simulink model "KP_sim"  (R2024b)
settings: Solver=VariableStepAuto  StartTime=0.0  StopTime=50  MaxStep=1e-3  RelTol=1e-3
values from neighbouring files (symbols this model uses):
  A = amplitudeValues(amplitudeIndex)    [KP_grid_results_generation.m]
  frequencyHz = frequencyValues(frequencyIndex)    [KP_grid_results_generation.m]
  x0 = [initialAngle; initialAngularVelocity]    [KP_grid_results_generation.m]
settings Model: Creator=Pedro  LastModifiedBy=Pedro

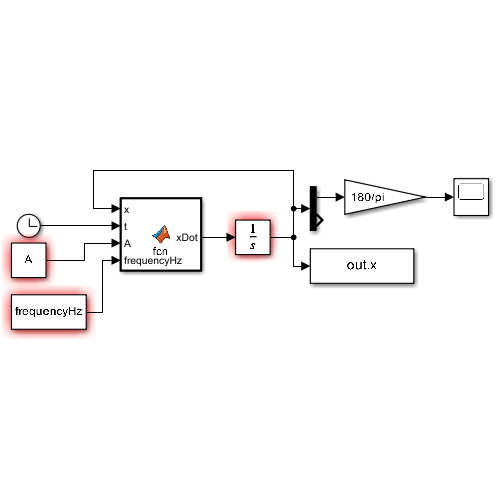
[thumbnail: Simulink's stored preview of the top-level diagram]
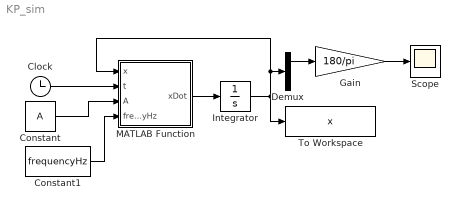
== system KP_sim ==
  Clock : Clock
  Constant : Constant  Value=A
  Constant1 : Constant  Value=frequencyHz
  Demux : Demux  Outputs=2
  Gain : Gain  Gain=180/pi
  Integrator : Integrator  InitialCondition=x0
  MATLAB Function : MATLAB Function  TreatAsAtomicUnit=on
  Scope : Scope
  To Workspace : ToWorkspace  VariableName=x  SaveFormat=Timeseries  SampleTime=-1
  wires:
  MATLAB Function/1(xDot) -> Integrator/1
  Integrator/1 -> MATLAB Function/1(x), Demux/1, To Workspace/1
  Clock/1 -> MATLAB Function/2(t)
  Gain/1 -> Scope/1
  Demux/1 -> Gain/1
  Constant/1 -> MATLAB Function/3(A)
  Constant1/1 -> MATLAB Function/4(frequencyHz)

== matlab function KP_sim/MATLAB Function ==
  data: x input; xDot output; t input; A input; frequencyHz input
function xDot = fcn(x,t,A,frequencyHz)

% Physical parameters
g = 9.81;       % gravitational acceleration [m/s^2]
L = 1.0;        % pendulum length [m]
zeta = 0.01;    % damping ratio [-]

% Natural and excitation frequencies
Omega = sqrt(g/L);
omega = 2*pi*frequencyHz;

% Base acceleration amplitude
% A is the base displacement amplitude [m]
a0 = A*omega^2;

% Periodic excitation
phi = cos(omega*t);

% States
theta = x(1);
thetaDot = x(2);

% Nonlinear inverted-pendulum equation
thetaDDot = -2*zeta*Omega*thetaDot ...
    - (-Omega^2 + (a0/L)*phi)*sin(theta);

% State derivative
xDot = [thetaDot; thetaDDot];

end
